simulink model "robot_arm_plant"  (R2025a)
settings: Solver=ode4  StartTime=0.0  StopTime=2.0  FixedStep=Ts_plant  RelTol=1e-3
settings Model: Creator=yk  LastModifiedBy=yk

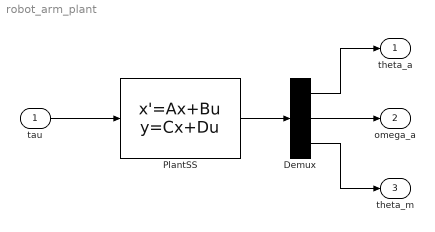
== system robot_arm_plant ==
  tau : Inport
  Demux : Demux  Outputs=3
  PlantSS : StateSpace  A=[0 1 0 0;-29610 -15 29610 5;0 0 0 1;5922 1 -5922 -5]  B=[0;1000;0;0]  C=[0 0 1 0;0 0 0 1;1 0 0 0]  D=[0;0;0]  InitialCondition=0
  theta_a : Outport
  omega_a : Outport  Port=2
  theta_m : Outport  Port=3
  wires:
  tau/1 -> PlantSS/1
  PlantSS/1 -> Demux/1
  Demux/1 -> theta_a/1
  Demux/2 -> omega_a/1
  Demux/3 -> theta_m/1
